simulink model "MatlabServerTCPIPModel"  (R2016a)
settings: Solver=VariableStepAuto  StartTime=0.0  StopTime=inf  RelTol=1e-3
settings Model: Creator=kalkadry  LastModifiedBy=kalkadry

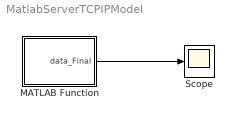
== system MatlabServerTCPIPModel ==
  MATLAB Function : MATLAB Function  TreatAsAtomicUnit=on
  Scope : Scope
  wires:
  MATLAB Function/1(data_Final) -> Scope/1

== matlab function MatlabServerTCPIPModel/MATLAB Function ==
  data: data_Final output
function  data_Final = fcn()
%#codegen

data_Final = zeros(64,1);
coder.extrinsic('tcpip');

% Accept a connection from any machine on port 30000.
t = tcpip('0.0.0.0', 30000, 'NetworkRole', 'server');

%Open a connection. This will not return until a connection is received.
fopen(t);

% Get client data
data = get(t,'BytesAvailable');

data_Final = fread(t, data);
